simulink model "Moteur_Partiel_Meca"  (Simulink 7.9)
settings: Solver=ode45  StartTime=0.0  StopTime=T_Sim  RelTol=1e-3
values from neighbouring files (symbols this model uses):
  Den_Meca = [Jeq/fv 1]    [BE_Chaines.m]    (also in Param_Moteur.m)
  K_C1 = RRoue*(R1/R2)*M*g*(pi/180)/n    (= 0.145534279678)    [BE_Chaines.m]    (also in Param_Moteur.m)
  KI = 76e-3    (= 0.076)    [BE_Chaines.m]    (also in Param_Moteur.m)
  Num_Meca = 1/fv    (= 4000)    [BE_Chaines.m]    (also in Param_Moteur.m)
settings Model: Creator=trocache  LastModifiedBy=trocache

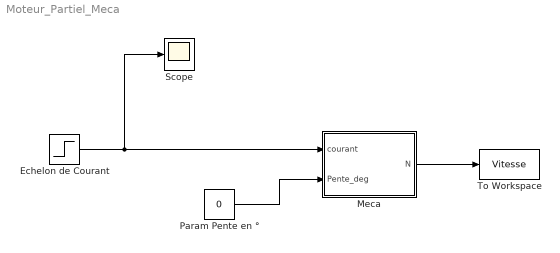
== system Moteur_Partiel_Meca ==
  Echelon de Courant : Step  Time=0.00  After=10  SampleTime=0
  Meca : Subsystem
  Param Pente en ° : Constant  Value=0
  Scope : Scope
  To Workspace : ToWorkspace  VariableName=Vitesse  SampleTime=-1  SaveFormat=Structure With Time
  wires:
  Param Pente en °/1 -> Meca/2(Pente_deg)
  Echelon de Courant/1 -> Scope/1, Meca/1(courant)
  Meca/1(N) -> To Workspace/1

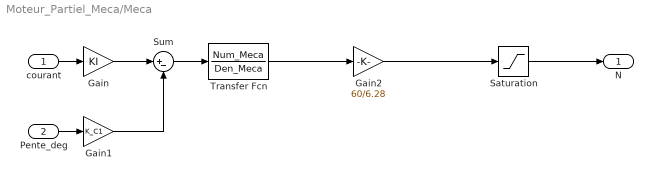
== system Moteur_Partiel_Meca/Meca ==
  courant : Inport
  Pente_deg : Inport  Port=2
  Gain : Gain  Gain=KI
  Gain1 : Gain  Gain=K_C1
  Gain2 : Gain  Gain=60/6.28
  Saturation : Saturate  UpperLimit=3000  LowerLimit=-3000
  Sum : Sum  Inputs=|+-
  Transfer Fcn : TransferFcn  Numerator=Num_Meca  Denominator=Den_Meca
  N : Outport
  wires:
  Sum/1 -> Transfer Fcn/1
  Gain/1 -> Sum/1
  courant/1 -> Gain/1
  Transfer Fcn/1 -> Gain2/1
  Pente_deg/1 -> Gain1/1
  Gain1/1 -> Sum/2
  Gain2/1 -> Saturation/1
  Saturation/1 -> N/1
